simulink model "LDW_mask"  (Simulink 7.8)
settings: Solver=FixedStepDiscrete  StartTime=0.0  StopTime=10.0  FixedStep=1/100  RelTol=1e-3
undefined symbols (not defined in the file or in its folder): High, num_targets, slselsubs
libraries: simulink x35, dspmtrx3 x13, visiontextngfix x9, dspsigops x6, simulink_extras x4, visiontransforms x4, dspstat3 x4, dspswit3 x3, dspadpt3 x3, dspindex x2, visionconversions x2, visionstatistics x2
(part 1 of 3)
settings Model: Creator=MarcinB  LastModifiedBy=Krzysztof
settings OptimizationCC: InlineParams=on
settings DebuggingCC: ParameterPrecisionLossMsg=none  FcnCallInpInsideContextMsg=Use local settings  FrameProcessingCompatibilityMsg=error
settings SFSimCC: SimParseCustomCode=off
settings CodeAppCC: CustomSymbolStrType=$N$R$M_T

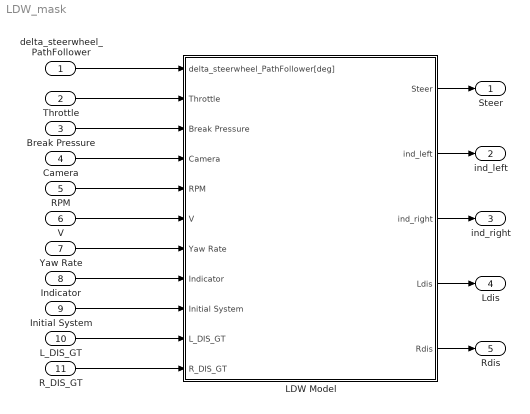
== system LDW_mask ==
  delta_steerwheel_PathFollower : Inport
  Throttle : Inport  Port=2
  Break Pressure : Inport  Port=3
  Camera : Inport  Port=4
  RPM : Inport  Port=5
  V : Inport  Port=6
  Yaw Rate : Inport  Port=7
  Indicator : Inport  Port=8
  Initial System : Inport  Port=9
  L_DIS_GT : Inport  Port=10
  R_DIS_GT : Inport  Port=11
  LDW Model : Subsystem  InitFcn=|  mask(Lane Keep Assistance System){imgSize=[375 500], LKAGfactor=1.3, cfq1=50, efq1=100, GUI_Switch=on, Plots_Switch=on, gfq1=25, Video_Switch=on, FVideo_Switch=on, vfq1=25}
      | % Image size                                                               
      | imgSize = [375 500];                                                       
      |                                                                            
      | % Number of rows and columns in the image region to process.               
      | numRows = floor(imgSize(1)/1.76);                                          
      | numCols = imgSize(2);                                                      
      |                                                                            
      | % To handle different video sizes other than [240 360], scaling the Hough  
      | % transform rho values by the below factor is required.                    
      | factor = sqrt(sum(imgSize.^2)) / sqrt(sum([240 360].^2));                  
      |                                                                            
      | %% parameters for the second lane                                          
      | %approximately 35:45 (0-based index: 414:424)                              
      | startIdxRho_R = floor(factor * 414);                                       
      | NumRhos_R = floor(factor * 11);                                            
      |                                                                            
      | %approximately -90:-70 degrees (0-based index: 0:20)                       
      | startIdxTheta_R = 0;                                                       
      | NumThetas_R = 21;                                                          
      | neighborhood_R =  [min(7,NumRhos_R), min(7,NumThetas_R)];                  
      |                                                                            
      | %approximately 379:415 (0-based index: 0:35)                               
      | startIdxRho_L = floor(factor * 379);                                       
      | NumRhos_L = floor(factor * 36);                                            
      |                                                                            
      | %approximately 55:85 degrees (0-based index: 145: 175)                     
      | startIdxTheta_L = 145;                                                     
      | NumThetas_L = 21;                                                          
      | neighborhood_L =  [min(7,NumRhos_L), min(7,NumThetas_L)];                  
      |                                                                            
      | % Maximum number of lanes to find in the current frame.(2)                 
      | expLaneNum = 2;                                                            
      |                                                                            
      | % Maximum number of lanes to store in the tracking repository.             
      | maxLaneNum = 20;                                                           
      |                                                                            
      | % Angular resolution of Hough transform, i.e., the width of a theta bin is 
      | % pi/angleNum. 180                                                         
      | angleNum = 180;                                                            
      |                                                                            
      | % Maximum allowable change of lane distance metric between two frames.(75) 
      | trackThreshold = 75;                                                       
      |                                                                            
      | % Minimum number of frames a lane must be detected to become a valid lane. 
      | frameFound = 5;                                                            
      |                                                                            
      | % Maximum number of frames a lane can be missed without marking it invalid.
      | frameLost = 20;                                                            
      |                                                                            
      | % Size of the neighborhood around the maxima over which the Hough          
      | % transforms values are suppressed. (Used in Find Local Maxima block)      
      | neighborhood = [101, 151];                                                 
      |                                                                            
      | % Distance threshold for lane crossing warning; valid range is (0, 0.5).   
      | thrWarn = 0.3;                                                             
      |                                                                            
      | % Weight (tweaking factor) of the angular difference for calculating the   
      | % distance metric between two lanes. It is typically chosen to be close    
      | % to the input image rows.                                                 
      | distanceMetricWeight = 375;%350;                                           
      |                                                                            
      | % Audio track used for lane cross warning.                                 
      | load viprumbling.mat;
      mask prompts: imgSize "Image size [pxls]"; LKAGfactor "LKA Assist reaction 1.0-1.5 (1.3)[-]"; cfq1 "Camera frequency [Hz]"; efq1 "Compilation Sheet frequency [Hz]"; GUI_Switch "EGO State GUI"; Plots_Switch "Plots of distance to line Error"; gfq1 "EGO State GUI frequency [Hz]"; Video_Switch "Video Result"; FVideo_Switch "Filtred Video Output"; vfq1 "Video Result frequency [Hz]"
      mask init:
      | %Maximum number of lanes to find in the current frame.(2) 
      | expLaneNum=1;
      | %Maximum number of lanes to store in the tracking repository.
      | maxLaneNum=4;
      | %maxLaneNum=20;
      | %Angular resolution of Hough transform, i.e., the width of a theta bin is pi/angleNum. 180
      | angleNum=180;
      | %Maximum allowable change of lane distance metric between two frames.(75)
      | trackThreshold=75;
      | %Minimum number of frames a lane must be detected to become a valid lane.
      | frameFound=3;
      | %frameFound=5;
      | %Maximum number of frames a lane can be missed without marking it invalid
      | frameLost=200;
      | %frameLost=20;
      | %Size of the neighborhood around the maxima over which the Hough 101 151
      | neighborhood=[101, 151];
      | %neighborhood=[301, 81];
      | %Distance threshold for lane crossing warning; valid range is (0, 0.5)
      | thrWarn=0.3;
      | %thrWarn=0.4;
      | thrWarn1=0.3;
      | %Weight (tweaking factor) of the angular difference for calculating the distance <br>  metric between two lanes. It is typically chosen to be close to the input image rows.
      | distanceMetricWeight=375;
      | %distanceMetricWeight=200;
      | 
      | cfq=1/cfq1;
      | efq=1/efq1;
      | vfq=1/vfq1;
      | gfq=1/gfq1;
      | %numRows = floor(imgSize(1)/1.35)-10; %(1.76)
      | numRows = 245; %240
      | numCols = imgSize(2);
      | imgRows=imgSize(1)-numRows;
      | factor = sqrt(sum(imgSize.^2)) / sqrt(sum([240 360].^2));
      | %factor = 1;
      | startIdxRho_R = floor(factor * 414);
      | %startIdxRho_R = 414;
      | NumRhos_R = floor(factor * 11);
      | %NumRhos_R = 11;
      | startIdxTheta_R = 0;
      | NumThetas_R = 21;
      | neighborhood_R =  [min(7,NumRhos_R), min(7,NumThetas_R)];
      | %neighborhood_R =  [7 7];
      | startIdxRho_L = floor(factor * 379);
      | %startIdxRho_L = 379;
      | NumRhos_L = floor(factor * 36);
      | %NumRhos_L= 36;
      | startIdxTheta_L = 145;
      | NumThetas_L = 21;
      | neighborhood_L =  [min(7,NumRhos_L), min(7,NumThetas_L)];
      | %neighborhood_L = [7 7];
      | corner = [zeros(ceil((imgSize(1) - numRows - 21)*0.3)), ones(ceil((imgSize(1) - numRows - 21)*0.3), floor(imgSize(2)*0.6 - (imgSize(1) - numRows - 21)*0.3)); ones(ceil((imgSize(1) - numRows - 21)*0.7), round(imgSize(2)*0.6))];
      mask CallbackString:
      | ||||en = get_param(gcb,'MaskEnables');
      | a = get_param(gcb, 'GUI_Switch');
      | b = get_param(gcb, 'Plots_Switch');
      | if or(strcmp(a,'on'),strcmp(b,'on'))
      |     en{7} = 'on';
      | else
      |     en{7} = 'off';
      | end
      | set_param(gcb,'MaskEnables',en);|en = get_param(gcb,'MaskEnables');
      | a = get_param(gcb, 'GUI_Switch');
      | b = get_param(gcb, 'Plots_Switch');
      | if or(strcmp(a,'on'),strcmp(b,'on'))
      |     en{7} = 'on';
      | else
      |     en{7} = 'off';
      | end
      | set_param(gcb,'MaskEnables',en);
      | 
      | 
      |     ||en = get_param(gcb,'MaskEnables');
      | c = get_param(gcb, 'Video_Switch');
      | d = get_param(gcb, 'FVideo_Switch');
      | if or(strcmp(c,'on'),strcmp(d,'on'))
      |     en{10} = 'on';
      | else
      |     en{10} = 'off';
      | end
      | set_param(gcb,'MaskEnables',en);|en = get_param(gcb,'MaskEnables');
      | c = get_param(gcb, 'Video_Switch');
      | d = get_param(gcb, 'FVideo_Switch');
      | if or(strcmp(c,'on'),strcmp(d,'on'))
      |     en{10} = 'on';
      | else
      |     en{10} = 'off';
      | end
      | set_param(gcb,'MaskEnables',en);|
  Steer : Outport
  ind_left : Outport  Port=2
  ind_right : Outport  Port=3
  Ldis : Outport  Port=4
  Rdis : Outport  Port=5
  wires:
  delta_steerwheel_PathFollower/1 -> LDW Model/1(delta_steerwheel_PathFollower[deg])
  Throttle/1 -> LDW Model/2(Throttle)
  Break Pressure/1 -> LDW Model/3(Break Pressure)
  Camera/1 -> LDW Model/4(Camera)
  RPM/1 -> LDW Model/5(RPM)
  LDW Model/1(Steer) -> Steer/1
  V/1 -> LDW Model/6(V)
  Indicator/1 -> LDW Model/8(Indicator)
  Yaw Rate/1 -> LDW Model/7(Yaw Rate)
  Initial System/1 -> LDW Model/9(Initial System)
  L_DIS_GT/1 -> LDW Model/10(L_DIS_GT)
  R_DIS_GT/1 -> LDW Model/11(R_DIS_GT)
  LDW Model/2(ind_left) -> ind_left/1
  LDW Model/3(ind_right) -> ind_right/1
  LDW Model/4(Ldis) -> Ldis/1
  LDW Model/5(Rdis) -> Rdis/1

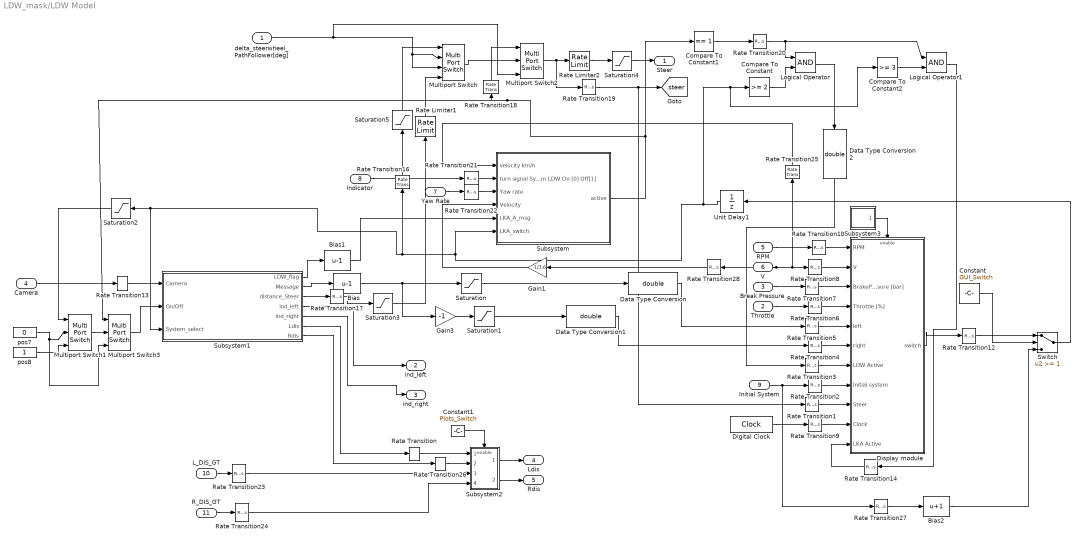
== system LDW_mask/LDW Model ==
  delta_steerwheel_PathFollower[deg] : Inport
  Throttle : Inport  Port=2  SampleTime=efq
  Break Pressure : Inport  Port=3  SampleTime=efq
  Camera : Inport  Port=4  OutDataTypeStr=uint8  SampleTime=cfq
  RPM : Inport  Port=5  SampleTime=efq
  V : Inport  Port=6  SampleTime=efq
  Yaw Rate : Inport  Port=7  SampleTime=efq
  Indicator : Inport  Port=8  OutDataTypeStr=uint8  SampleTime=efq
  Initial System : Inport  Port=9  SampleTime=efq
  L_DIS_GT : Inport  Port=10  SampleTime=efq
  R_DIS_GT : Inport  Port=11  SampleTime=efq
  Bias : Bias  Bias=-1
  Bias1 : Bias  Bias=-1
  Bias2 : Bias  Bias=1
  Compare To Constant : simulink/Logic and Bit Operations/Compare To Constant  relop=>=  const=2  OutDataTypeStr=uint8
  Compare To Constant1 : simulink/Logic and Bit Operations/Compare To Constant  relop===  const=1  OutDataTypeStr=uint8
  Compare To Constant2 : simulink/Logic and Bit Operations/Compare To Constant  relop=>=  const=3  OutDataTypeStr=uint8
  Constant : Constant  Value=GUI_Switch  SampleTime=cfq
  Constant1 : Constant  Value=Plots_Switch  SampleTime=gfq
  Data Type Conversion : DataTypeConversion  OutDataTypeStr=double  SampleTime=cfq
  Data Type Conversion1 : DataTypeConversion  OutDataTypeStr=double
  Data Type Conversion2 : DataTypeConversion  OutDataTypeStr=double
  Digital Clock : DigitalClock  SampleTime=0.01
  Display module : Subsystem
      mask init:
      | % Maximum value of brake pressure [bar]
      | MaxBrakePressure = 150;
  Gain1 : Gain  Gain=1/3.6
  Gain3 : Gain  Gain=-1
  Logical Operator : Logic  AllPortsSameDT=off  OutDataTypeStr=boolean  SampleTime=cfq
  Logical Operator1 : Logic  AllPortsSameDT=off  OutDataTypeStr=boolean  SampleTime=cfq
  Multiport Switch : MultiPortSwitch  zeroidx=off
  Multiport Switch1 : MultiPortSwitch  Inputs=2  zeroidx=off
  Multiport Switch2 : MultiPortSwitch  Inputs=2  zeroidx=off
  Multiport Switch3 : MultiPortSwitch  Inputs=2  zeroidx=off  SampleTime=cfq
  Rate Limiter1 : RateLimiter  RisingSlewLimit=540  FallingSlewLimit=-540  SampleTimeMode=inherited
  Rate Limiter2 : RateLimiter  RisingSlewLimit=720  FallingSlewLimit=-720  SampleTimeMode=inherited
  Rate Transition{,1..10,14,23..24,26} (15 alike) : RateTransition  OutPortSampleTime=gfq
  Rate Transition{12,19..22,25,27..28} (8 alike) : RateTransition  OutPortSampleTime=cfq
  Rate Transition13 : RateTransition  X0=1  OutPortSampleTime=cfq
  Rate Transition16 : RateTransition  X0=1  OutPortSampleTime=efq
  Rate Transition17 : RateTransition  OutPortSampleTime=efq
  Rate Transition18 : RateTransition  X0=1  OutPortSampleTime=efq
  Saturation : Saturate  UpperLimit=1  LowerLimit=0
  Saturation1 : Saturate  UpperLimit=1  LowerLimit=0
  Saturation2 : Saturate  UpperLimit=2  LowerLimit=1
  Saturation3 : Saturate  UpperLimit=200  LowerLimit=-200
  Saturation4 : Saturate  UpperLimit=720  LowerLimit=-720
  Saturation5 : Saturate  UpperLimit=3  LowerLimit=1
  Subsystem : Subsystem
  Subsystem1 : Subsystem
  Subsystem2 : Subsystem
  Subsystem3 : Subsystem
  Switch : Switch  Threshold=1
  Unit Delay1 : UnitDelay  X0=2  SampleTime=cfq
  pos7 : Constant  Tag=pos  Value=0  SampleTime=cfq
  pos8 : Constant  Tag=pos  SampleTime=cfq
  Steer : Outport
  ind_left : Outport  Port=2
  ind_right : Outport  Port=3
  Ldis : Outport  Port=4
  Rdis : Outport  Port=5
  tag scope: steer=global
  wires:
  Indicator/1 -> Rate Transition21/1
  Throttle/1 -> Rate Transition6/1
  Camera/1 -> Rate Transition13/1
  Break Pressure/1 -> Rate Transition7/1
  Multiport Switch1/1 -> Multiport Switch3/2
  Subsystem/1(active) -> Multiport Switch3/1, Rate Transition18/1, Compare To Constant1/1
  Multiport Switch/1 -> Multiport Switch2/2
  pos7/1 -> Multiport Switch3/3, Multiport Switch1/2
  Multiport Switch2/1 -> Rate Transition19/1, Rate Limiter2/1
  Saturation2/1 -> Multiport Switch1/1
  Data Type Conversion1/1 -> Rate Transition4/1
  Data Type Conversion/1 -> Rate Transition5/1
  Saturation1/1 -> Data Type Conversion1/1
  Saturation/1 -> Data Type Conversion/1
  Gain3/1 -> Saturation1/1
  V/1 -> Rate Transition8/1, Rate Transition25/1, Rate Transition28/1
  RPM/1 -> Rate Transition10/1
  delta_steerwheel_PathFollower[deg]/1 -> Multiport Switch/3, Multiport Switch/2, Multiport Switch2/3
  pos8/1 -> Multiport Switch1/3
  Bias1/1 -> Subsystem/5(LKA_A_msg)
  Bias/1 -> Saturation/1, Gain3/1
  Unit Delay1/1 -> Rate Transition16/1, Saturation2/1, Subsystem1/3(System_select), Subsystem/6(LKA_switch), Compare To Constant/1, Compare To Constant2/1
  Compare To Constant1/1 -> Rate Transition20/1
  Compare To Constant/1 -> Logical Operator/2
  Logical Operator/1 -> Data Type Conversion2/1
  Data Type Conversion2/1 -> Rate Transition3/1
  Yaw Rate/1 -> Rate Transition22/1
  Gain1/1 -> Subsystem/4(Velocity)
  Initial System/1 -> Rate Transition2/1, Rate Transition27/1
  Saturation3/1 -> Rate Limiter1/1
  Saturation4/1 -> Steer/1
  L_DIS_GT/1 -> Rate Transition23/1
  R_DIS_GT/1 -> Rate Transition24/1
  Constant/1 -> Switch/2
  Digital Clock/1 -> Rate Transition9/1
  Rate Transition9/1 -> Display module/10(Clock)
  Rate Transition1/1 -> Display module/9(Steer)
  Rate Transition2/1 -> Display module/8(Initial system)
  Rate Transition3/1 -> Display module/7(LDW Active)
  Rate Transition4/1 -> Display module/6(right)
  Rate Transition5/1 -> Display module/5(left)
  Rate Transition6/1 -> Display module/4(Throttle [%])
  Rate Transition7/1 -> Display module/3(BrakePressure [bar])
  Rate Transition8/1 -> Display module/2(V)
  Rate Transition10/1 -> Display module/1(RPM)
  Subsystem3/1(Out1) -> Display module/Enable
  Rate Transition16/1 -> Saturation5/1
  Rate Transition18/1 -> Multiport Switch2/1
  Rate Transition19/1 -> [steer], Rate Transition1/1
  Rate Transition20/1 -> Logical Operator/1, Logical Operator1/1
  Rate Transition23/1 -> Subsystem2/3(L_DIS_GT)
  Rate Transition24/1 -> Subsystem2/4(R_DIS_GT)
  Saturation5/1 -> Multiport Switch/1
  Rate Transition17/1 -> Saturation3/1
  Rate Limiter2/1 -> Saturation4/1
  Bias2/1 -> Switch/3
  Switch/1 -> Unit Delay1/1
  Rate Transition27/1 -> Bias2/1
  Display module/1(switch) -> Rate Transition12/1
  Rate Transition12/1 -> Switch/1
  Rate Transition21/1 -> Subsystem/2(turn signal System LDW On [0] Off[1])
  Rate Transition22/1 -> Subsystem/3(Yaw rate)
  Rate Transition25/1 -> Subsystem/1(velocity km/h)
  Rate Transition28/1 -> Gain1/1
  Subsystem1/5(ind_right) -> ind_right/1
  Subsystem1/4(ind_left) -> ind_left/1
  Subsystem1/1(LDW_flag) -> Bias1/1
  Subsystem1/2(Message) -> Bias/1
  Subsystem1/3(distance_Steer) -> Rate Transition17/1
  Multiport Switch3/1 -> Subsystem1/2(On/Off)
  Compare To Constant2/1 -> Logical Operator1/2
  Logical Operator1/1 -> Rate Transition14/1
  Rate Transition14/1 -> Display module/11(LKA Active)
  Rate Transition13/1 -> Subsystem1/1(Camera)
  Constant1/1 -> Subsystem2/Enable
  Rate Transition/1 -> Subsystem2/1(Ldis)
  Rate Transition26/1 -> Subsystem2/2(Rdis)
  Subsystem1/6(Ldis) -> Rate Transition/1
  Subsystem1/7(Rdis) -> Rate Transition26/1
  Subsystem2/1(Ldis1) -> Ldis/1
  Subsystem2/2(Rdis1) -> Rdis/1
  Rate Limiter1/1 -> Multiport Switch/4

== system LDW_mask/LDW Model/Display module ==
  RPM : Inport
  V : Inport  Port=2
  BrakePressure [bar] : Inport  Port=3
  Throttle [%] : Inport  Port=4
  left : Inport  Port=5
  right : Inport  Port=6
  LDW Active : Inport  Port=7
  Initial system : Inport  Port=8
  Steer : Inport  Port=9
  Clock : Inport  Port=10
  LKA Active : Inport  Port=11
  Enable : EnablePort  StatesWhenEnabling=reset
  Brake Pressure [bar] : Gain  Gain=100/MaxBrakePressure
  DISPLAY : M-S-Function  FunctionName=msfcn_PlotSpeed  Parameters=GUI_Switch cfq
      mask Display:
      | port_label('input',1,'RPM');
      | port_label('input',2,'V');
      | port_label('input',3,'BrakePress');
      | port_label('input',4,'Throttle');
      | port_label('input',5,'left');
      | port_label('input',6,'right');
      | port_label('input',7,'LDW Active');
      | port_label('input',8,'Initial system');
      | port_label('input',9,'Steer');
      | port_label('input',10,'Clock');
      | port_label('input',11,'LKA Active');
      | port_label('output',1,'Switch')
  Data Type Conversion : DataTypeConversion
  Gain2 : Gain  Gain=1/2
  Rounding Function{,1..3} (4 alike) : Rounding  Operator=round
  Saturation : Saturate  UpperLimit=3  LowerLimit=1
  switch : Outport
  wires:
  Initial system/1 -> DISPLAY/8
  LDW Active/1 -> DISPLAY/7
  Saturation/1 -> switch/1
  DISPLAY/1 -> Saturation/1
  right/1 -> DISPLAY/6
  V/1 -> Rounding Function1/1
  RPM/1 -> Rounding Function/1
  left/1 -> DISPLAY/5
  Throttle [%]/1 -> Rounding Function3/1
  BrakePressure [bar]/1 -> Brake Pressure [bar]/1
  Brake Pressure [bar]/1 -> Rounding Function2/1
  Rounding Function3/1 -> DISPLAY/4
  Rounding Function2/1 -> DISPLAY/3
  Rounding Function1/1 -> DISPLAY/2
  Rounding Function/1 -> DISPLAY/1
  Steer/1 -> Gain2/1
  Data Type Conversion/1 -> DISPLAY/9
  Gain2/1 -> Data Type Conversion/1
  Clock/1 -> DISPLAY/10
  LKA Active/1 -> DISPLAY/11

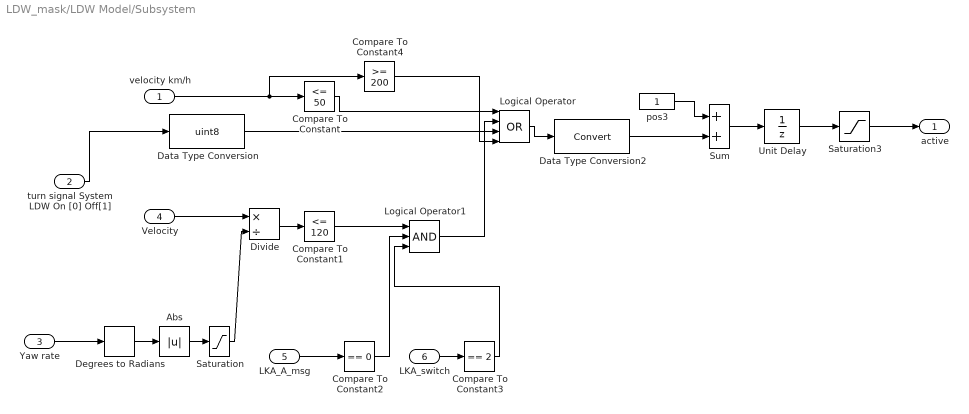
== system LDW_mask/LDW Model/Subsystem ==
  velocity km/h : Inport
  turn signal System LDW On [0] Off[1] : Inport  Port=2
  Yaw rate : Inport  Port=3
  Velocity : Inport  Port=4
  LKA_A_msg : Inport  Port=5
  LKA_switch : Inport  Port=6
  Abs : Abs
  Compare To Constant : simulink/Logic and Bit Operations/Compare To Constant  relop=<=  const=50  OutDataTypeStr=uint8
  Compare To Constant1 : simulink/Logic and Bit Operations/Compare To Constant  relop=<=  const=120  OutDataTypeStr=uint8
  Compare To Constant2 : simulink/Logic and Bit Operations/Compare To Constant  relop===  const=0  OutDataTypeStr=uint8
  Compare To Constant3 : simulink/Logic and Bit Operations/Compare To Constant  relop===  const=2  OutDataTypeStr=uint8
  Compare To Constant4 : simulink/Logic and Bit Operations/Compare To Constant  relop=>=  const=200  OutDataTypeStr=uint8
  Data Type Conversion : DataTypeConversion  OutDataTypeStr=uint8
  Data Type Conversion2 : DataTypeConversion
  Degrees to Radians : simulink_extras/Transformations/Degrees to Radians
  Divide : Product  Inputs=*/
  Logical Operator : Logic  Operator=OR  Inputs=4  AllPortsSameDT=off  OutDataTypeStr=boolean
  Logical Operator1 : Logic  Inputs=3  AllPortsSameDT=off  OutDataTypeStr=boolean
  Saturation : Saturate  UpperLimit=inf  LowerLimit=0.001
  Saturation3 : Saturate  UpperLimit=2  LowerLimit=1
  Sum : Sum
  Unit Delay : UnitDelay  X0=1  SampleTime=-1
  pos3 : Constant  Tag=pos
  active : Outport
  wires:
  Saturation3/1 -> active/1
  Unit Delay/1 -> Saturation3/1
  Sum/1 -> Unit Delay/1
  turn signal System LDW On [0] Off[1]/1 -> Data Type Conversion/1
  velocity km/h/1 -> Compare To Constant/1, Compare To Constant4/1
  Data Type Conversion2/1 -> Sum/2
  Logical Operator/1 -> Data Type Conversion2/1
  Compare To Constant/1 -> Logical Operator/1
  pos3/1 -> Sum/1
  Divide/1 -> Compare To Constant1/1
  Velocity/1 -> Divide/1
  Yaw rate/1 -> Degrees to Radians/1
  Abs/1 -> Saturation/1
  Degrees to Radians/1 -> Abs/1
  Saturation/1 -> Divide/2
  Data Type Conversion/1 -> Logical Operator/2
  Compare To Constant1/1 -> Logical Operator1/1
  Logical Operator1/1 -> Logical Operator/3
  Compare To Constant2/1 -> Logical Operator1/2
  LKA_A_msg/1 -> Compare To Constant2/1
  LKA_switch/1 -> Compare To Constant3/1
  Compare To Constant3/1 -> Logical Operator1/3
  Compare To Constant4/1 -> Logical Operator/4

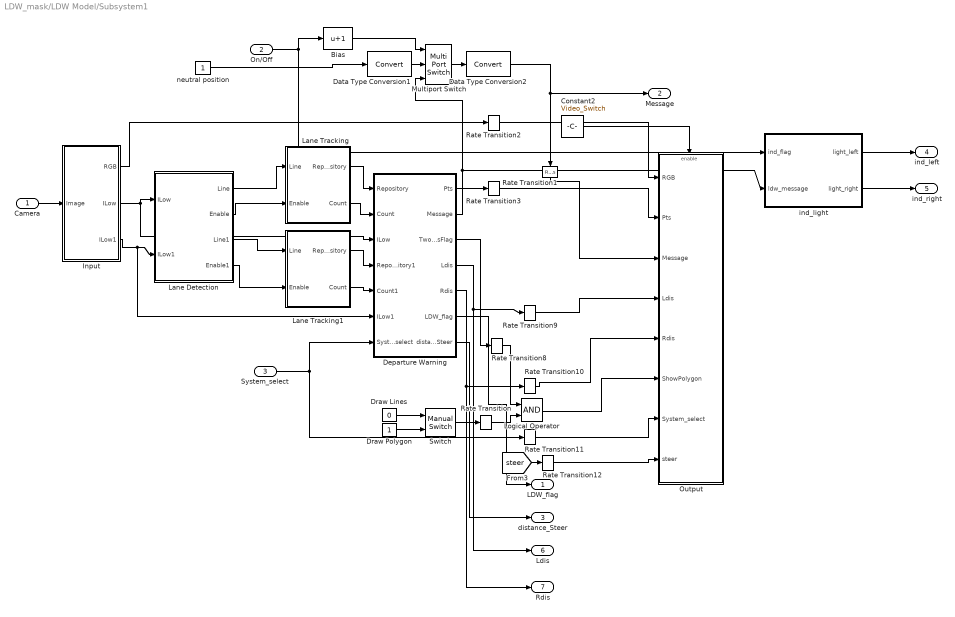
== system LDW_mask/LDW Model/Subsystem1 ==
  Camera : Inport  OutDataTypeStr=uint8  PortDimensions=imgSize
  On/Off : Inport  Port=2
  System_select : Inport  Port=3
  Bias : Bias  Bias=1
  Constant2 : Constant  Value=Video_Switch  SampleTime=vfq
  Data Type Conversion1 : DataTypeConversion
  Data Type Conversion2 : DataTypeConversion
  Departure Warning : Subsystem
  Draw Lines : Constant  Value=0  VectorParams1D=off  OutDataTypeStr=boolean  SampleTime=efq
  Draw Polygon : Constant  VectorParams1D=off  OutDataTypeStr=boolean  SampleTime=efq
  Input : Subsystem
  Lane Detection : Subsystem
  Lane Tracking : Subsystem
  Lane Tracking1 : Subsystem
  Logical Operator : Logic  AllPortsSameDT=off  OutDataTypeStr=boolean  SampleTime=vfq
  Multiport Switch : MultiPortSwitch  Inputs=2  zeroidx=off  SampleTime=cfq
  Output : Subsystem
  Rate Transition{,1..3,8..12} (9 alike) : RateTransition  OutPortSampleTime=vfq
  Switch : simulink/Signal Routing/Manual Switch  sw=0  action=0  varsize=off
  ind_light : Subsystem  mask{Ts_ind=efq}
      mask prompts: Ts_ind "Indicator Sample Time"
  neutral position : Constant  VectorParams1D=off  OutDataTypeStr=int8  SampleTime=cfq
  LDW_flag : Outport
  Message : Outport  Port=2
  distance_Steer : Outport  Port=3
  ind_left : Outport  Port=4
  ind_right : Outport  Port=5
  Ldis : Outport  Port=6
  Rdis : Outport  Port=7
  wires:
  Lane Detection/1(Line) -> Lane Tracking/1(Line)
  Lane Detection/2(Enable) -> Lane Tracking/2(Enable)
  Lane Tracking/1(Repository) -> Departure Warning/1(Repository)
  Lane Tracking/2(Count) -> Departure Warning/2(Count)
  Input/1(RGB) -> Rate Transition2/1
  Departure Warning/1(Pts) -> Rate Transition3/1
  Draw Lines/1 -> Switch/1
  Draw Polygon/1 -> Switch/2
  Departure Warning/3(TwoLanesFlag) -> Rate Transition8/1
  Switch/1 -> Rate Transition/1
  Logical Operator/1 -> Output/6(ShowPolygon)
  Input/2(ILow) -> Lane Detection/1(ILow), Departure Warning/3(ILow)
  Camera/1 -> Input/1(Image)
  Lane Detection/3(Line1) -> Lane Tracking1/1(Line)
  Lane Detection/4(Enable1) -> Lane Tracking1/2(Enable)
  Input/3(ILow1) -> Departure Warning/6(ILow1), Lane Detection/2(ILow1)
  Lane Tracking1/1(Repository) -> Departure Warning/4(Repository1)
  Lane Tracking1/2(Count) -> Departure Warning/5(Count1)
  Departure Warning/4(Ldis) -> Rate Transition9/1, Ldis/1
  Departure Warning/5(Rdis) -> Rate Transition10/1, Rdis/1
  Departure Warning/6(LDW_flag) -> LDW_flag/1
  Departure Warning/7(distance_Steer) -> distance_Steer/1
  ind_light/1(light_left) -> ind_left/1
  ind_light/2(light_right) -> ind_right/1
  System_select/1 -> Departure Warning/7(System_select), Rate Transition11/1
  Data Type Conversion1/1 -> Multiport Switch/2
  Bias/1 -> Multiport Switch/1
  On/Off/1 -> Bias/1, ind_light/1(ind_flag)
  neutral position/1 -> Data Type Conversion1/1
  Multiport Switch/1 -> Data Type Conversion2/1
  Data Type Conversion2/1 -> Message/1, Rate Transition1/1
  Departure Warning/2(Message) -> Multiport Switch/3, ind_light/2(ldw_message)
  Constant2/1 -> Output/Enable
  Rate Transition/1 -> Logical Operator/2
  Rate Transition1/1 -> Output/3(Message)
  Rate Transition2/1 -> Output/1(RGB)
  Rate Transition3/1 -> Output/2(Pts)
  Rate Transition8/1 -> Logical Operator/1
  Rate Transition9/1 -> Output/4(Ldis)
  Rate Transition10/1 -> Output/5(Rdis)
  Rate Transition11/1 -> Output/7(System_select)
  [steer] -> Rate Transition12/1
  Rate Transition12/1 -> Output/8(steer)

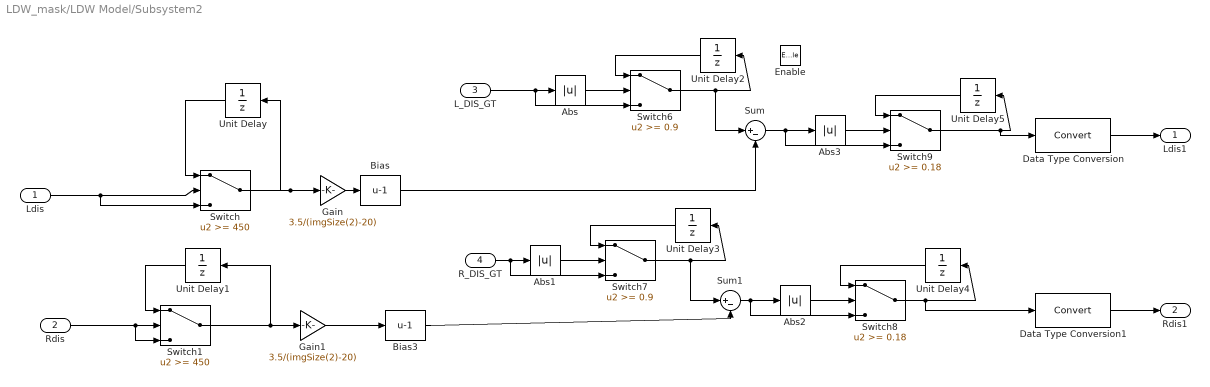
== system LDW_mask/LDW Model/Subsystem2 ==
  Ldis : Inport
  Rdis : Inport  Port=2
  L_DIS_GT : Inport  Port=3
  R_DIS_GT : Inport  Port=4
  Enable : EnablePort
  Abs{,1..3} (4 alike) : Abs
  Bias : Bias  Bias=-1
  Bias3 : Bias  Bias=-1
  Data Type Conversion : DataTypeConversion
  Data Type Conversion1 : DataTypeConversion
  Gain : Gain  Gain=3.5/(imgSize(2)-20)  OutDataTypeStr=double
  Gain1 : Gain  Gain=3.5/(imgSize(2)-20)  OutDataTypeStr=double
  Sum : Sum  Inputs=|+-
  Sum1 : Sum  Inputs=|+-
  Switch : Switch  Threshold=450
  Switch1 : Switch  Threshold=450
  Switch6 : Switch  Threshold=0.9
  Switch7 : Switch  Threshold=0.9
  Switch8 : Switch  Threshold=0.18
  Switch9 : Switch  Threshold=0.18
  Unit Delay{,1..5} (6 alike) : UnitDelay  SampleTime=-1
  Ldis1 : Outport
  Rdis1 : Outport  Port=2
  wires:
  Rdis/1 -> Switch1/2, Switch1/3
  Unit Delay1/1 -> Switch1/1
  Switch1/1 -> Gain1/1, Unit Delay1/1
  Gain1/1 -> Bias3/1
  Gain/1 -> Bias/1
  Ldis/1 -> Switch/2, Switch/3
  Unit Delay/1 -> Switch/1
  Switch/1 -> Gain/1, Unit Delay/1
  Data Type Conversion1/1 -> Rdis1/1
  Data Type Conversion/1 -> Ldis1/1
  Sum/1 -> Switch9/3, Abs3/1
  Abs3/1 -> Switch9/2
  Switch9/1 -> Data Type Conversion/1, Unit Delay5/1
  Unit Delay5/1 -> Switch9/1
  Sum1/1 -> Switch8/3, Abs2/1
  Abs2/1 -> Switch8/2
  Switch8/1 -> Data Type Conversion1/1, Unit Delay4/1
  Unit Delay4/1 -> Switch8/1
  R_DIS_GT/1 -> Switch7/3, Abs1/1
  Abs1/1 -> Switch7/2
  Switch7/1 -> Unit Delay3/1, Sum1/1
  Unit Delay3/1 -> Switch7/1
  Abs/1 -> Switch6/2
  Switch6/1 -> Unit Delay2/1, Sum/1
  L_DIS_GT/1 -> Switch6/3, Abs/1
  Unit Delay2/1 -> Switch6/1
  Bias3/1 -> Sum1/2
  Bias/1 -> Sum/2

== system LDW_mask/LDW Model/Subsystem3 ==
  Constant2 : Constant  Value=GUI_Switch  SampleTime=cfq
  Rate Transition : RateTransition  Integrity=off  OutPortSampleTime=gfq
  Out1 : Outport
  wires:
  Constant2/1 -> Rate Transition/1
  Rate Transition/1 -> Out1/1

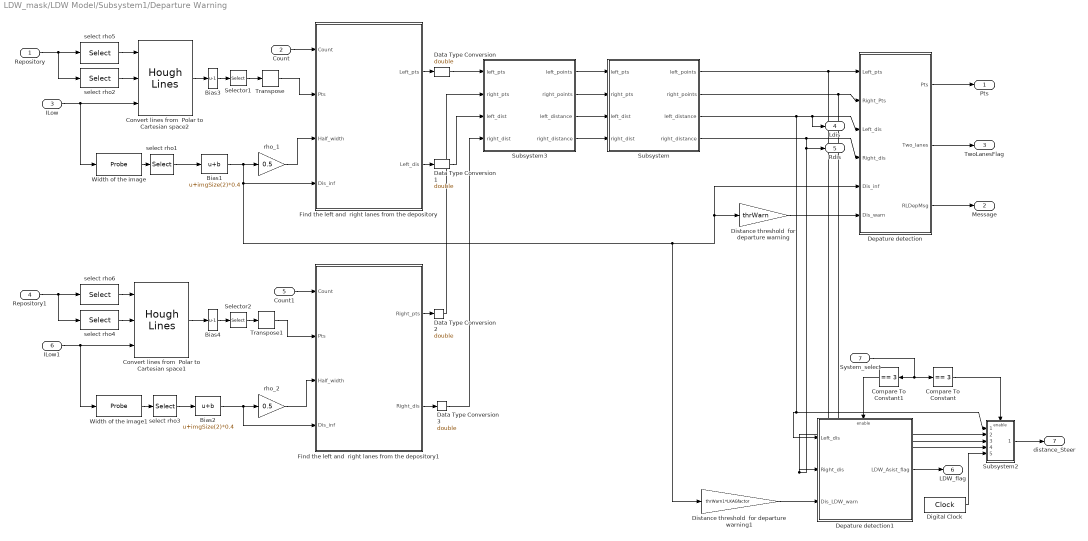
== system LDW_mask/LDW Model/Subsystem1/Departure Warning ==
  Repository : Inport
  Count : Inport  Port=2
  ILow : Inport  Port=3
  Repository1 : Inport  Port=4
  Count1 : Inport  Port=5
  ILow1 : Inport  Port=6
  System_select : Inport  Port=7
  Bias1 : Bias  Bias=imgSize(2)*0.4
  Bias2 : Bias  Bias=imgSize(2)*0.4
  Bias3 : Bias  Bias=-1
  Bias4 : Bias  Bias=-1
  Compare To Constant : simulink/Logic and Bit Operations/Compare To Constant  relop===  const=3  OutDataTypeStr=uint8
  Compare To Constant1 : simulink/Logic and Bit Operations/Compare To Constant  relop===  const=3  OutDataTypeStr=uint8
  Convert lines from  Polar to Cartesian space1 : visiontransforms/Hough Lines  sineCompMethod=Trigonometric function  thetaRes=pi/180  firstCoeffMode=Specify word length  firstCoeffWordLength=16  firstCoeffFracLength=15  prodOutputMode=Binary point scaling  prodOutputWordLength=32  prodOutputFracLength=16  roundingMode=Nearest  overflowMode=on
  Convert lines from  Polar to Cartesian space2 : visiontransforms/Hough Lines  sineCompMethod=Trigonometric function  thetaRes=pi/180  firstCoeffMode=Specify word length  firstCoeffWordLength=16  firstCoeffFracLength=15  prodOutputMode=Binary point scaling  prodOutputWordLength=32  prodOutputFracLength=16  roundingMode=Nearest  overflowMode=on
  Data Type Conversion{,1..3} (4 alike) : DataTypeConversion  OutDataTypeStr=double
  Depature detection : Subsystem
  Depature detection1 : Subsystem
  Digital Clock : DigitalClock  SampleTime=cfq
  Distance threshold  for departure warning : Gain  Gain=thrWarn  OutDataTypeStr=Inherit: Same as input
  Distance threshold  for departure warning1 : Gain  Gain=thrWarn1*LKAGfactor  OutDataTypeStr=Inherit: Same as input
  Find the left and  right lanes from the depository : Subsystem  TreatAsAtomicUnit=on
  Find the left and  right lanes from the depository1 : Subsystem  TreatAsAtomicUnit=on
  Selector1 : Selector  NumberOfDimensions=2  InputPortWidth=3  IndexOptions=Select all,Index vector (dialog)  Indices=[2 1],[2 1 4 3]  OutputSizes=1,1
  Selector2 : Selector  NumberOfDimensions=2  InputPortWidth=3  IndexOptions=Select all,Index vector (dialog)  Indices=[2 1],[2 1 4 3]  OutputSizes=1,1
  Subsystem : Subsystem  mask{limit_down=140, limit_up=170}
      mask prompts: limit_down "Limit down"; limit_up "Limit up"
  Subsystem2 : Subsystem
  Subsystem3 : Subsystem  mask{limit_down=130, limit_up=160}
      mask prompts: limit_down "Limit down"; limit_up "Limit up"
  Transpose : dspmtrx3/Transpose  Hermitian=off  overflowFlag=off
  Transpose1 : dspmtrx3/Transpose  Hermitian=off  overflowFlag=off
  Width of the image : Probe  ProbeWidth=off  ProbeSampleTime=off  ProbeComplexSignal=off  ProbeSignalDimensions=on  ProbeDimensionsDataType=int32
  Width of the image1 : Probe  ProbeWidth=off  ProbeSampleTime=off  ProbeComplexSignal=off  ProbeSignalDimensions=on  ProbeDimensionsDataType=int32
  rho_1 : Gain  Gain=0.5  OutDataTypeStr=Inherit: Same as input
  rho_2 : Gain  Gain=0.5  OutDataTypeStr=Inherit: Same as input
  select rho1 : Selector  InputPortWidth=2  IndexOptions=Index vector (dialog)  Indices=2  OutputSizes=1
  select rho2 : Selector  NumberOfDimensions=2  InputPortWidth=maxLaneNum  IndexOptions=Index vector (dialog),Select all  Indices=1,-1  OutputSizes=1
  select rho3 : Selector  InputPortWidth=2  IndexOptions=Index vector (dialog)  Indices=2  OutputSizes=1
  select rho4 : Selector  NumberOfDimensions=2  InputPortWidth=maxLaneNum  IndexOptions=Index vector (dialog),Select all  Indices=1,-1  OutputSizes=1
  select rho5 : Selector  NumberOfDimensions=2  InputPortWidth=maxLaneNum  IndexOptions=Index vector (dialog),Select all  Indices=2,-1  OutputSizes=1
  select rho6 : Selector  NumberOfDimensions=2  InputPortWidth=maxLaneNum  IndexOptions=Index vector (dialog),Select all  Indices=2,-1  OutputSizes=1
  Pts : Outport
  Message : Outport  Port=2
  TwoLanesFlag : Outport  Port=3
  Ldis : Outport  Port=4
  Rdis : Outport  Port=5
  LDW_flag : Outport  Port=6
  distance_Steer : Outport  Port=7
  wires:
  select rho2/1 -> Convert lines from  Polar to Cartesian space2/2
  Count/1 -> Find the left and  right lanes from the depository/1(Count)
  Repository/1 -> select rho5/1, select rho2/1
  select rho1/1 -> Bias1/1
  rho_1/1 -> Find the left and  right lanes from the depository/3(Half_width)
  Width of the image/1 -> select rho1/1
  Distance threshold  for departure warning/1 -> Depature detection/6(Dis_warn)
  Depature detection/1(Pts) -> Pts/1
  Depature detection/2(Two_lanes) -> TwoLanesFlag/1
  Depature detection/3(RLDepMsg) -> Message/1
  select rho5/1 -> Convert lines from  Polar to Cartesian space2/1
  Transpose1/1 -> Find the left and  right lanes from the depository1/2(Pts)
  select rho4/1 -> Convert lines from  Polar to Cartesian space1/2
  Count1/1 -> Find the left and  right lanes from the depository1/1(Count)
  Repository1/1 -> select rho4/1, select rho6/1
  ILow1/1 -> Convert lines from  Polar to Cartesian space1/3, Width of the image1/1
  select rho3/1 -> Bias2/1
  rho_2/1 -> Find the left and  right lanes from the depository1/3(Half_width)
  Width of the image1/1 -> select rho3/1
  select rho6/1 -> Convert lines from  Polar to Cartesian space1/1
  Find the left and  right lanes from the depository1/1(Right_pts) -> Data Type Conversion2/1
  Distance threshold  for departure warning1/1 -> Depature detection1/3(Dis_LDW_warn)
  Subsystem2/1(Out1) -> distance_Steer/1
  Digital Clock/1 -> Subsystem2/5(In5)
  Compare To Constant1/1 -> Depature detection1/Enable
  Depature detection1/1(LDW_Asist_flag) -> LDW_flag/1
  Compare To Constant/1 -> Subsystem2/Enable
  System_select/1 -> Compare To Constant1/1, Compare To Constant/1
  Bias1/1 -> rho_1/1, Find the left and  right lanes from the depository/4(Dis_inf), Distance threshold  for departure warning/1, Depature detection/5(Dis_inf), Distance threshold  for departure warning1/1
  Bias2/1 -> rho_2/1, Find the left and  right lanes from the depository1/4(Dis_inf)
  Subsystem3/1(left_points) -> Subsystem/1(left_pts)
  Subsystem3/2(right_points) -> Subsystem/2(right_pts)
  Subsystem3/3(left_distance) -> Subsystem/3(left_dist)
  Subsystem3/4(right_distance) -> Subsystem/4(right_dist)
  Find the left and  right lanes from the depository/1(Left_pts) -> Data Type Conversion/1
  Find the left and  right lanes from the depository/2(Left_dis) -> Data Type Conversion1/1
  Find the left and  right lanes from the depository1/2(Right_dis) -> Data Type Conversion3/1
  Subsystem/1(left_points) -> Depature detection/1(Left_pts), Subsystem2/3(In3)
  Subsystem/2(right_points) -> Depature detection/2(Right_Pts), Subsystem2/4(In4)
  Subsystem/3(left_distance) -> Depature detection1/1(Left_dis), Subsystem2/1(In1), Depature detection/3(Left_dis), Ldis/1
  Subsystem/4(right_distance) -> Rdis/1, Depature detection1/2(Right_dis), Subsystem2/2(In2), Depature detection/4(Right_dis)
  Data Type Conversion/1 -> Subsystem3/1(left_pts)
  Data Type Conversion1/1 -> Subsystem3/3(left_dist)
  Data Type Conversion2/1 -> Subsystem3/2(right_pts)
  Data Type Conversion3/1 -> Subsystem3/4(right_dist)
  ILow/1 -> Convert lines from  Polar to Cartesian space2/3, Width of the image/1
  Selector1/1 -> Transpose/1
  Bias3/1 -> Selector1/1
  Convert lines from  Polar to Cartesian space2/1 -> Bias3/1
  Transpose/1 -> Find the left and  right lanes from the depository/2(Pts)
  Selector2/1 -> Transpose1/1
  Bias4/1 -> Selector2/1
  Convert lines from  Polar to Cartesian space1/1 -> Bias4/1

== system LDW_mask/LDW Model/Subsystem1/Input ==
  note: For different video sizes, set imgSize appropriately in model
      | workspace and then press the "Reinitliaze from Source" button.
  Image : Inport
  2-D FIR Filter1 : visionfilter/2-D FIR Filter  separable=off  filtSrc=Specify via dialog  filterMtrx=[-1 0 1]  verticalFilter=[4 0]  horizontalFilter=[4 0]  outSize=Same as input port I  padType=Replicate  padSrc=Specify via dialog  padVal=0  method=Correlation  firstCoeffMode=Specify word length  firstCoeffWordLength=16  firstCoeffFracLength=14  firstCoeffSignedness=Signed  firstCoeffDataTypeStr=fixdt(1,16)  firstCoeffLastDataTypeStr=fixdt(1,16)  firstCoeffMin=[]  firstCoeffMax=[]  outputSignedness=Auto  outputMin=[]  outputMax=[]  accumDataTypeStr=Inherit: Same as product output  accumLastDataTypeStr=Inherit: Same as product output  prodOutputMode=Binary point scaling  prodOutputWordLength=32  prodOutputFracLength=10  prodOutputDataTypeStr=fixdt([],32,10)  prodOutputLastDataTypeStr=fixdt([],32,10)  roundingMode=Floor  overflowMode=on
  Clip image1 : dspmtrx3/Submatrix  RowSpan=All rows  RowStartMode=Index  RowStartIndex=numRows+1  RowEndMode=Offset from last  RowEndIndex=20  ColSpan=Range of columns  ColStartMode=First  ColStartIndex=1  ColEndMode=Offset from last  ColEndIndex=imgSize(2)*0.4
  Clip image2 : dspmtrx3/Submatrix  RowSpan=All rows  RowStartMode=Index  RowStartIndex=numRows+1  RowEndMode=Offset from last  RowEndIndex=20  ColSpan=Range of columns  ColStartMode=First  ColStartIndex=1  ColEndMode=Offset from last  ColEndIndex=imgSize(2)*0.4
  Clip image3 : dspmtrx3/Submatrix  RowSpan=Range of rows  RowStartMode=Index  RowStartIndex=numRows+1  RowEndMode=Offset from last  RowEndIndex=20  ColSpan=All columns  ColStartMode=First  ColStartIndex=1  ColEndMode=Offset from last  ColEndIndex=imgSize(2)*0.4
  Image Data Type Conversion : visionconversions/Image Data Type Conversion  outDT=single  isSigned=on  wordLen=16  numFracBits=0
  Image thresholding1 : visionconversions/Autothreshold  operator=>  threshOut=off  effMetricOut=off  userDefinedRange=off  umin=0  umax=255  outOfRngOpt=Warn and saturate  scaleThreshold=off  scaleFactor=1  P1Mode=Specify word length  P1WordLength=32  P1FracLength=30  P2Mode=Specify word length  P2WordLength=32  P2FracLength=22  P3Mode=Specify word length  P3WordLength=32  P3FracLength=14  P4Mode=Binary point scaling  P4WordLength=32  P4FracLength=15  Q1Mode=Specify word length  Q1WordLength=32  Q1FracLength=16  EMMode=Specify word length  EMWordLength=16  EMFracLength=14  roundingMode=Floor  overflowMode=off
  MATLAB Function : MATLAB Function  TreatAsAtomicUnit=on
  Matrix Concatenate : Concatenate  NumInputs=3  Mode=Multidimensional array  ConcatenateDimension=3
  Saturation1 : Saturate  UpperLimit=1  LowerLimit=0
  RGB : Outport
  ILow : Outport  Port=2
  ILow1 : Outport  Port=3
  wires:
  Image/1 -> Image Data Type Conversion/1
  Clip image2/1 -> ILow/1
  Image Data Type Conversion/1 -> Matrix Concatenate/2, Matrix Concatenate/1, Matrix Concatenate/3, Clip image3/1
  Matrix Concatenate/1 -> RGB/1
  MATLAB Function/1(y) -> Clip image1/1
  Clip image1/1 -> ILow1/1
  Saturation1/1 -> Image thresholding1/1
  2-D FIR Filter1/1 -> Saturation1/1
  Image thresholding1/1 -> Clip image2/1, MATLAB Function/1(u)
  Clip image3/1 -> 2-D FIR Filter1/1

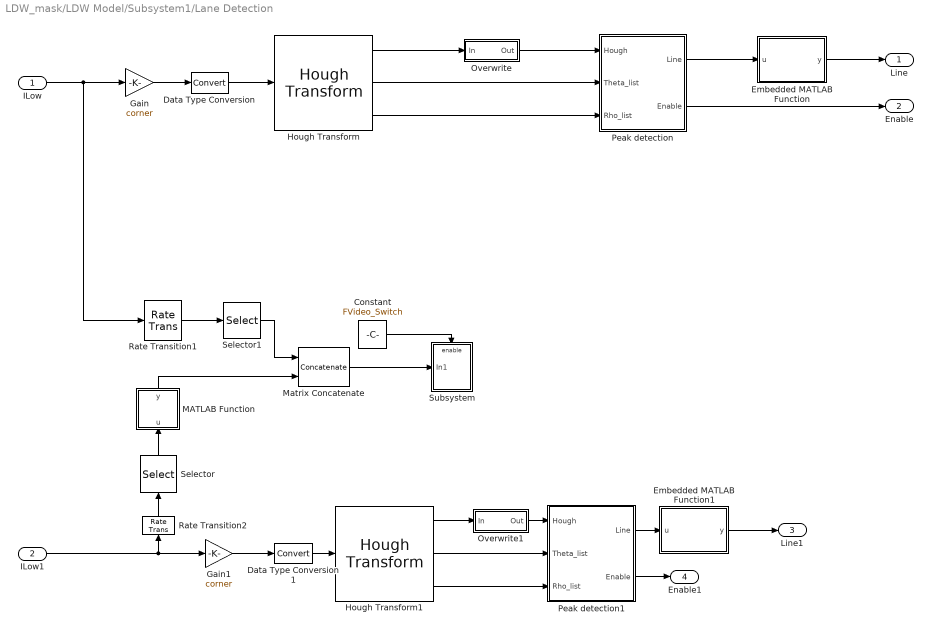
== system LDW_mask/LDW Model/Subsystem1/Lane Detection ==
  ILow : Inport
  ILow1 : Inport  Port=2
  Constant : Constant  Value=FVideo_Switch  SampleTime=vfq
  Data Type Conversion : DataTypeConversion
  Data Type Conversion1 : DataTypeConversion
  Embedded MATLAB Function : MATLAB Function  TreatAsAtomicUnit=on
  Embedded MATLAB Function1 : MATLAB Function  TreatAsAtomicUnit=on
  Gain : Gain  Gain=corner
  Gain1 : Gain  Gain=corner
  Hough Transform : visiontransforms/Hough Transform  theta_res=pi/angleNum  rho_res=1  out_theta_rho=on  outdtmode=single  firstCoeffMode=Binary point scaling  firstCoeffWordLength=16  firstCoeffFracLength=14  secondCoeffMode=Binary point scaling  secondCoeffWordLength=32  secondCoeffFracLength=16  outputMode=Binary point scaling  outputWordLength=16  outputFracLength=0  accumMode=Binary point scaling  accumWordLength=32  accumFracLength=20  prodOutputMode=Binary point scaling  prodOutputWordLength=32  prodOutputFracLength=20  memoryMode=Binary point scaling  memoryWordLength=32  memoryFracLength=16  roundingMode=Nearest  overflowMode=on
  Hough Transform1 : visiontransforms/Hough Transform  theta_res=pi/angleNum  rho_res=1  out_theta_rho=on  outdtmode=single  firstCoeffMode=Binary point scaling  firstCoeffWordLength=16  firstCoeffFracLength=14  secondCoeffMode=Binary point scaling  secondCoeffWordLength=32  secondCoeffFracLength=16  outputMode=Binary point scaling  outputWordLength=16  outputFracLength=0  accumMode=Binary point scaling  accumWordLength=32  accumFracLength=20  prodOutputMode=Binary point scaling  prodOutputWordLength=32  prodOutputFracLength=20  memoryMode=Binary point scaling  memoryWordLength=32  memoryFracLength=16  roundingMode=Nearest  overflowMode=on
  MATLAB Function : MATLAB Function  TreatAsAtomicUnit=on
  Matrix Concatenate : Concatenate  Mode=Multidimensional array  ConcatenateDimension=2
  Overwrite : Subsystem
  Overwrite1 : Subsystem
  Peak detection : Subsystem
  Peak detection1 : Subsystem
  Rate Transition1 : RateTransition  OutPortSampleTime=vfq
  Rate Transition2 : RateTransition  OutPortSampleTime=vfq
  Selector : Selector  NumberOfDimensions=2  InputPortWidth=3  IndexOptions=Select all,Index vector (dialog)  Indices=[1 3],1:imgSize(2)*0.5  OutputSizes=1,1
  Selector1 : Selector  NumberOfDimensions=2  InputPortWidth=3  IndexOptions=Select all,Index vector (dialog)  Indices=[1 3],1:imgSize(2)*0.5  OutputSizes=1,1
  Subsystem : Subsystem
  Line : Outport
  Enable : Outport  Port=2
  Line1 : Outport  Port=3
  Enable1 : Outport  Port=4
  wires:
  Overwrite/1(Out) -> Peak detection/1(Hough)
  Peak detection/2(Enable) -> Enable/1
  Peak detection/1(Line) -> Embedded MATLAB Function/1(u)
  Hough Transform/3 -> Peak detection/3(Rho_list)
  Hough Transform/2 -> Peak detection/2(Theta_list)
  Hough Transform/1 -> Overwrite/1(In)
  ILow/1 -> Gain/1, Rate Transition1/1
  Overwrite1/1(Out) -> Peak detection1/1(Hough)
  Peak detection1/2(Enable) -> Enable1/1
  Peak detection1/1(Line) -> Embedded MATLAB Function1/1(u)
  Hough Transform1/3 -> Peak detection1/3(Rho_list)
  Hough Transform1/2 -> Peak detection1/2(Theta_list)
  Hough Transform1/1 -> Overwrite1/1(In)
  ILow1/1 -> Gain1/1, Rate Transition2/1
  Gain/1 -> Data Type Conversion/1
  Gain1/1 -> Data Type Conversion1/1
  Data Type Conversion/1 -> Hough Transform/1
  Data Type Conversion1/1 -> Hough Transform1/1
  Embedded MATLAB Function/1(y) -> Line/1
  Embedded MATLAB Function1/1(y) -> Line1/1
  Rate Transition1/1 -> Selector1/1
  Constant/1 -> Subsystem/Enable
  Selector1/1 -> Matrix Concatenate/1
  Selector/1 -> MATLAB Function/1(u)
  Rate Transition2/1 -> Selector/1
  Matrix Concatenate/1 -> Subsystem/1(In1)
  MATLAB Function/1(y) -> Matrix Concatenate/2

== system LDW_mask/LDW Model/Subsystem1/Lane Tracking ==
  Line : Inport
  Enable : Inport  Port=2
  Kalman Filter : dspadpt3/Kalman Filter  num_targets=maxLaneNum  sourceEnable=Specify via input port <Enable>  isReset=on  X=zeros([4, 1])  P=100*eye(4)  A=[1 0 1 0;0 1 0 1; 0 0 1 0; 0 0 0 1]  sourceMeasure=Specify via Dialog  H=[1 0 0 0; 0 1 0 0]  Q=0.05*eye(4)  R=1*eye(2)  isOutputEstMeasure=on  isOutputEstState=off  isOutputEstError=off  isOutputPrdMeasure=on  isOutputPrdState=off  isOutputPrdError=off
  Matching : Subsystem
  Only update the lines which  Kalman filter has been  trained for enough time : simulink/Logic and Bit Operations/Compare To Constant  relop=>=  const=frameFound  OutDataTypeStr=boolean  ZeroCross=off
  Unit Delay : UnitDelay  X0=zeros(2,maxLaneNum)  SampleTime=-1
  Unit Delay1 : UnitDelay  SampleTime=-1
  Update : Subsystem  TreatAsAtomicUnit=on
  Repository : Outport
  Count : Outport  Port=2
  wires:
  Matching/2(Count) -> Only update the lines which  Kalman filter has been  trained for enough time/1, Unit Delay1/1, Count/1, Kalman Filter/2
  Only update the lines which  Kalman filter has been  trained for enough time/1 -> Update/3(Update)
  Unit Delay1/1 -> Matching/4(Count_ref)
  Unit Delay/1 -> Matching/3(Rep_ref)
  Line/1 -> Matching/1(Line)
  Enable/1 -> Matching/2(Enable)
  Matching/1(Repository) -> Update/1(Old), Kalman Filter/1
  Update/1(Out) -> Unit Delay/1
  Kalman Filter/2 -> Update/2(New)
  Kalman Filter/1 -> Repository/1

== system LDW_mask/LDW Model/Subsystem1/Lane Tracking1 ==
  Line : Inport
  Enable : Inport  Port=2
  Kalman Filter : dspadpt3/Kalman Filter  num_targets=maxLaneNum  sourceEnable=Specify via input port <Enable>  isReset=on  X=zeros([4, 1])  P=100*eye(4)  A=[1 0 1 0;0 1 0 1; 0 0 1 0; 0 0 0 1]  sourceMeasure=Specify via Dialog  H=[1 0 0 0; 0 1 0 0]  Q=0.05*eye(4)  R=1*eye(2)  isOutputEstMeasure=on  isOutputEstState=off  isOutputEstError=off  isOutputPrdMeasure=on  isOutputPrdState=off  isOutputPrdError=off
  Matching : Subsystem
  Only update the lines which  Kalman filter has been  trained for enough time : simulink/Logic and Bit Operations/Compare To Constant  relop=>=  const=frameFound  OutDataTypeStr=boolean  ZeroCross=off
  Unit Delay : UnitDelay  X0=zeros(2,maxLaneNum)  SampleTime=-1
  Unit Delay1 : UnitDelay  SampleTime=-1
  Update : Subsystem  TreatAsAtomicUnit=on
  Repository : Outport
  Count : Outport  Port=2
  wires:
  Kalman Filter/1 -> Repository/1
  Kalman Filter/2 -> Update/2(New)
  Update/1(Out) -> Unit Delay/1
  Matching/1(Repository) -> Kalman Filter/1, Update/1(Old)
  Enable/1 -> Matching/2(Enable)
  Line/1 -> Matching/1(Line)
  Unit Delay/1 -> Matching/3(Rep_ref)
  Unit Delay1/1 -> Matching/4(Count_ref)
  Only update the lines which  Kalman filter has been  trained for enough time/1 -> Update/3(Update)
  Matching/2(Count) -> Kalman Filter/2, Count/1, Unit Delay1/1, Only update the lines which  Kalman filter has been  trained for enough time/1
